simulink model "MRAC"  (R2022b)
settings: Solver=FixedStepAuto  StartTime=0.0  StopTime=40  FixedStep=0.01  RelTol=1e-3
values from neighbouring files (symbols this model uses):
  Ks = 195    [Servo_calc_lq.m]    (also in Servo_calc_lq_d.m; servo_start.m)
  Ts = 0.86    [Servo_calc_lq.m]    (also in Servo_calc_lq_d.m; servo_start.m)
settings Model: Creator=artur  LastModifiedBy=artur

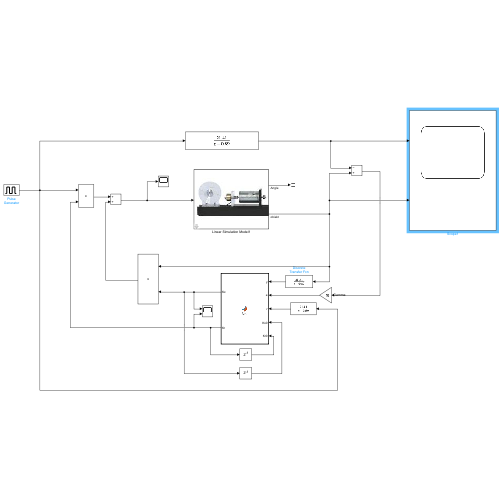
[thumbnail: Simulink's stored preview of the top-level diagram]
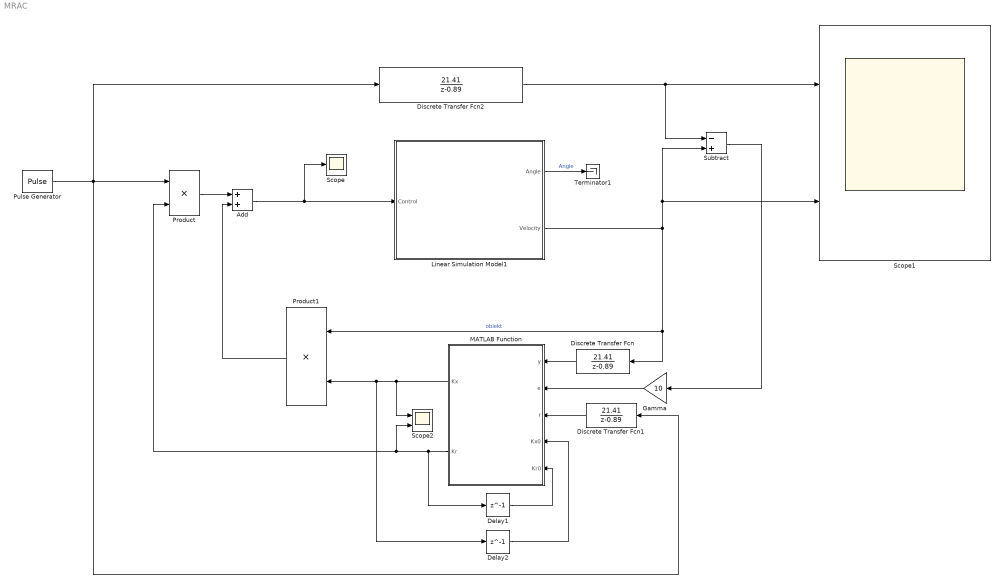
== system MRAC ==
  Add : Sum
  Delay1 : Delay  DelayLength=1  InitialCondition=0
  Delay2 : Delay  DelayLength=1  InitialCondition=0
  Discrete Transfer Fcn : DiscreteTransferFcn  Numerator=[21.41]  Denominator=[1 -0.89]
  Discrete Transfer Fcn1 : DiscreteTransferFcn  Numerator=[21.41]  Denominator=[1 -0.89]
  Discrete Transfer Fcn2 : DiscreteTransferFcn  Numerator=[21.41]  Denominator=[1 -0.89]
  Gamma : Gain  Gain=10
  Linear Simulation Model1 : Subsystem  mask{x0=[0 0]}
      mask prompts: x0 "Initial conditions [angle vel]"
      mask Display: image(imread('Servo_m.JPG'))
  MATLAB Function : MATLAB Function  TreatAsAtomicUnit=on
  Product : Product
  Product1 : Product
  Pulse Generator : DiscretePulseGenerator  PulseType=Time based  Period=10  PulseWidth=50
  Scope : Scope
  Scope1 : Scope  NumInputPorts=2
  Scope2 : Scope  NumInputPorts=2
  Subtract : Sum  Inputs=-+
  Terminator1 : Terminator
  wires:
  Linear Simulation Model1/1(Angle) -> Terminator1/1  "Angle"
  Discrete Transfer Fcn2/1 -> Scope1/1, Subtract/1
  Product/1 -> Add/1
  Add/1 -> Scope/1, Linear Simulation Model1/1(Control)
  Product1/1 -> Add/2
  MATLAB Function/1(Kx) -> Scope2/1, Delay2/1, Product1/2
  Linear Simulation Model1/2(Velocity) -> Subtract/2, Scope1/2, Discrete Transfer Fcn/1, Product1/1  "obiekt"
  Subtract/1 -> Gamma/1
  Delay1/1 -> MATLAB Function/5(Kr0)
  Delay2/1 -> MATLAB Function/4(Kx0)
  Pulse Generator/1 -> Discrete Transfer Fcn2/1, Discrete Transfer Fcn1/1, Product/1
  MATLAB Function/2(Kr) -> Delay1/1, Product/2, Scope2/2
  Discrete Transfer Fcn1/1 -> MATLAB Function/3(r)
  Discrete Transfer Fcn/1 -> MATLAB Function/1(y)
  Gamma/1 -> MATLAB Function/2(e)

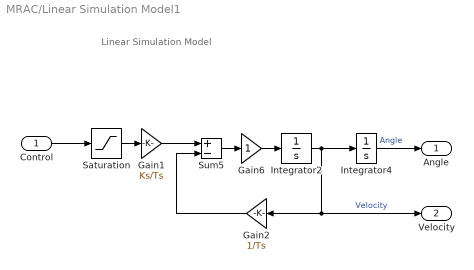
== system MRAC/Linear Simulation Model1 ==
  note: Linear Simulation Model
  Control : Inport
  Gain1 : Gain  Gain=Ks/Ts  SaturateOnIntegerOverflow=on  OutDataTypeStr=Inherit: Same as input  ParamDataTypeStr=Inherit: Same as input
  Gain2 : Gain  Gain=1/Ts  SaturateOnIntegerOverflow=on  OutDataTypeStr=Inherit: Same as input  ParamDataTypeStr=Inherit: Same as input
  Gain6 : Gain  SaturateOnIntegerOverflow=on  OutDataTypeStr=Inherit: Same as input  ParamDataTypeStr=Inherit: Same as input
  Integrator2 : Integrator  InitialCondition=x0(2)
  Integrator4 : Integrator  InitialCondition=x0(1)
  Saturation : Saturate  UpperLimit=1  LowerLimit=-1
  Sum5 : Sum  Inputs=+-  InputSameDT=on  SaturateOnIntegerOverflow=on  OutDataTypeStr=Inherit: Same as first input
  Angle : Outport  InitialOutput=0  VectorParamsAs1DForOutWhenUnconnected=off
  Velocity : Outport  Port=2  InitialOutput=0  VectorParamsAs1DForOutWhenUnconnected=off
  wires:
  Sum5/1 -> Gain6/1
  Gain2/1 -> Sum5/2
  Integrator2/1 -> Integrator4/1, Velocity/1, Gain2/1  "Velocity"
  Integrator4/1 -> Angle/1  "Angle"
  Gain6/1 -> Integrator2/1
  Control/1 -> Saturation/1
  Saturation/1 -> Gain1/1
  Gain1/1 -> Sum5/1

== matlab function MRAC/MATLAB Function ==
  data: y input; e input; r input; Kx0 input; Kr0 input; Kx output; Kr output
function [Kx, Kr] = fcn(y,e,r,Kx0,Kr0)


Kr = Kr0 + e * r;
Kx = Kx0 - e * y;
